simulink model "lsys6_1"  (R2020b)
settings: Solver=VariableStepAuto  StartTime=0.0  StopTime=20  RelTol=1e-3
settings Model: Creator=반달  LastModifiedBy=반달
settings DataIOCC: ReturnWorkspaceOutputs=off

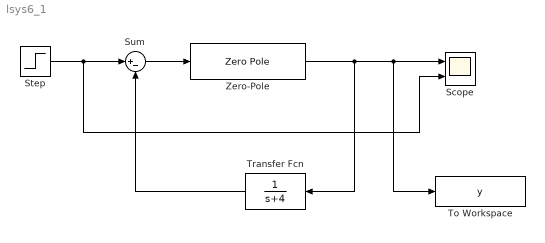
== system lsys6_1 ==
  Scope : Scope  NumInputPorts=2
  Step : Step  Time=3  SampleTime=0
  Sum : Sum  Inputs=|+-
  To Workspace : ToWorkspace  VariableName=y  SaveFormat=Structure With Time  SampleTime=-1
  Transfer Fcn : TransferFcn  Denominator=[1 4]
  Zero-Pole : ZeroPole  Zeros=[1 3]  Poles=[0 -2 -3]  Gain=2
  wires:
  Step/1 -> Sum/1, Scope/2
  Sum/1 -> Zero-Pole/1
  Zero-Pole/1 -> Transfer Fcn/1, To Workspace/1, Scope/1
  Transfer Fcn/1 -> Sum/2
